simulink model "model1"  (R2023a)
settings: Solver=ode4  StartTime=0.0  StopTime=500  FixedStep=simulation_dt  RelTol=1e-3
undefined symbols (not defined in the file or in its folder): input, k_harmonics, magnitude, simulation_dt
libraries: simulink x3
settings Model: Creator=dionl  LastModifiedBy=dionl

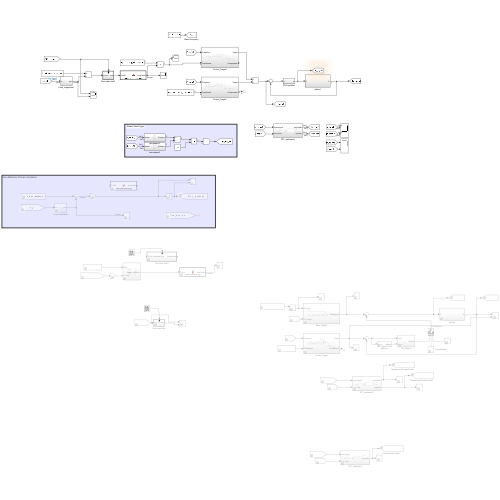
[thumbnail: Simulink's stored preview of the top-level diagram]
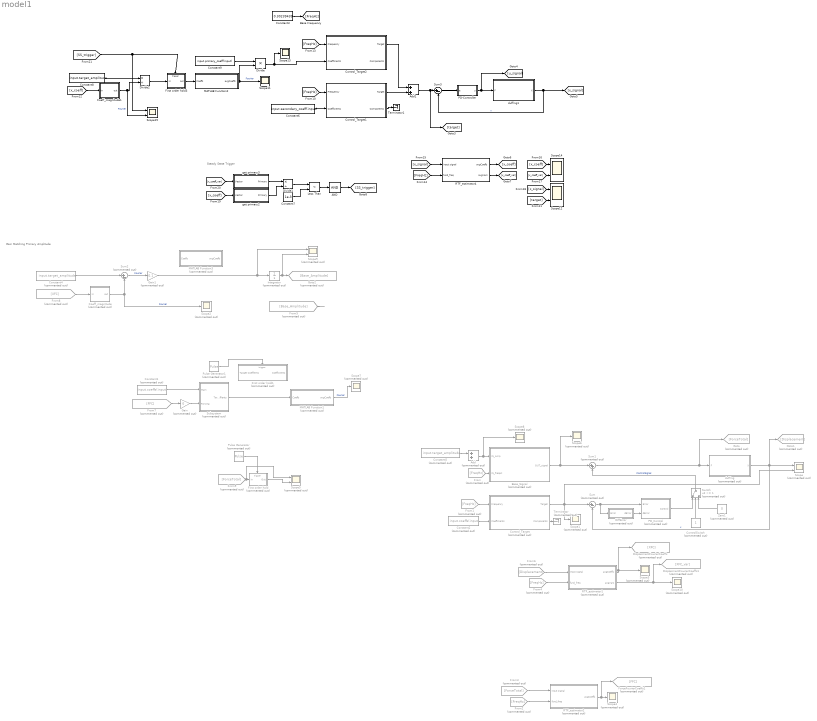
== system model1 ==
  note: Steady State Trigger
  note: Gain Matching Primary Amplitude
  AND : Logic  Inputs=1  IconShape=distinctive  AllPortsSameDT=off  OutDataTypeStr=boolean
  Add : Sum  Commented=on
  Add1 : Sum
  Base_Signal : Subsystem  Commented=on
  Coeff_magnitude : Subsystem  Commented=on
  Coeff_magnitude1 : Subsystem
  Constant1 : Constant  Commented=on  Value=input.coeffs(input)
  Constant2 : Constant  Commented=on  Value=input.coeffs(input)
  Constant3 : Constant  Value=0.30239439
  Constant4 : Constant  Commented=on  Value=input.target_amplitude
  Constant5 : Constant  Commented=on  Value=input.target_amplitude
  Constant6 : Constant  Value=input.secondary_coeff(input)
  Constant7 : Constant  Value=1e-3
  Constant8 : Constant  Value=input.target_amplitude
  Constant9 : Constant  Value=input.primary_coeff(input)
  ControlSwitch : Constant  Commented=on
  Control_Target : Subsystem  Commented=on
  Control_Target1 : Subsystem
  Control_Target2 : Subsystem
  DiffError : Subsystem  Commented=on
  DisplacmentFourierCoeffs : Goto  Commented=on  GotoTag=XFC
  DisplacmentFourierCoeffs1 : Goto  Commented=on  GotoTag=XFC_var
  Divide : Product  Inputs=**
  Divide1 : Product  Inputs=*/
  Divide2 : Product  Inputs=*/
  First order hold : Subsystem  Commented=on  TreatAsAtomicUnit=on
  First order hold1 : Subsystem  Commented=on  TreatAsAtomicUnit=on
  First order hold3 : Subsystem  TreatAsAtomicUnit=on
  ForceFourierCoeffs1 : Goto  Commented=on  GotoTag=FFC
  From{,1..2,4} (4 alike) : From  Commented=on  GotoTag=FreqHz
  From3 : From  Commented=on  GotoTag=ForceTotal
  From5 : From  Commented=on  GotoTag=Base_Amplitude
  From6 : From  Commented=on  GotoTag=Displacement
  From7 : From  Commented=on  GotoTag=FFC
  From8 : From  Commented=on  GotoTag=XFC
  From9 : From  Commented=on  GotoTag=ForceTotal
  Gain : Gain  Commented=on  Gain=0
  Gain1 : Gain  Commented=on  Gain=0.1
  Goto : Goto  Commented=on  GotoTag=ForceTotal
  Goto1 : Goto  Commented=on  GotoTag=Displacement
  Goto2 : Goto  Commented=on  GotoTag=Base_Amplitude
  Integrator : Integrator  Commented=on
  Less Than : RelationalOperator  Operator=<  OutDataTypeStr=boolean  RndMeth=Simplest  InputSameDT=off
  MATLAB Function1 : MATLAB Function  Commented=on  TreatAsAtomicUnit=on
  MATLAB Function2 : MATLAB Function  TreatAsAtomicUnit=on
  MATLAB Function3 : MATLAB Function  Commented=on  TreatAsAtomicUnit=on
  PD-Controller : Subsystem
  PD_Control : Subsystem  Commented=on
  Pulse Generator : DiscretePulseGenerator  Commented=on  PulseType=Time based  Period=1  PulseWidth=5
  Pulse Generator1 : DiscretePulseGenerator  Commented=on  PulseType=Time based  Period=100  PulseWidth=5  PhaseDelay=simulation_dt
  RTF_estimator1 : Subsystem  Commented=on
  RTF_estimator2 : Subsystem  Commented=on
  RTF_estimator4 : Subsystem
  Scope : Scope  Commented=on  NumInputPorts=2
  Scope{1..4,6..8,10} (8 alike) : Scope  Commented=on
  Scope11 : Scope
  Scope12 : Scope  NumInputPorts=2
  Scope13 : Scope
  Scope14 : Scope  NumInputPorts=2
  Scope15 : Scope  NumInputPorts=2
  Scope5 : Scope  Commented=on  NumInputPorts=2
  Scope9 : Scope  Commented=on  NumInputPorts=2
  Subsystem : Subsystem  Commented=on
  Sum : Sum  Commented=on  Inputs=|+-
  Sum1 : Sum  Commented=on  Inputs=|++
  Sum2 : Sum  Commented=on  Inputs=|+-
  Sum3 : Sum  Inputs=|+-
  Switch : Switch  Commented=on  Threshold=1  SaturateOnIntegerOverflow=off  InputSameDT=off
  Terminator : Terminator  Commented=on
  Terminator1 : Terminator
  Zero1 : Constant  Commented=on  Value=0
  duffing : Subsystem  Commented=on
  duffing1 : Subsystem
  get primary2 : Subsystem
  get primary3 : Subsystem
  wires:
  From/1 -> Base_Signal/2(IN_freqHz)
  Base_Signal/1(OUT_signal) -> Scope6/1, Sum1/1
  Control_Target/1(Target) -> Scope1/1, Scope/2, Sum/1
  duffing/1(X) -> Goto1/1, Scope/1, Sum/2  "x"
  Sum/1 -> DiffError/1(Error), PD_Control/1(Error)
  DiffError/1(dError) -> PD_Control/2(dError)
  Switch/1 -> Sum1/2  "ControlSignal"
  ControlSwitch/1 -> Switch/2
  Zero1/1 -> Switch/3
  PD_Control/1(Control) -> Switch/1
  Sum1/1 -> Goto/1, duffing/1(F)
  Constant3/1 -> [FreqHz]
  From1/1 -> Control_Target/1(Frequency)
  From4/1 -> RTF_estimator1/2(fund_freq)
  RTF_estimator1/1(avgCoeffs) -> Scope3/1, DisplacmentFourierCoeffs/1
  RTF_estimator2/1(avgCoeffs) -> ForceFourierCoeffs1/1, Scope4/1
  From2/1 -> RTF_estimator2/2(fund_freq)
  From3/1 -> RTF_estimator2/1(input signal)
  Control_Target/2(Components) -> Terminator/1
  From6/1 -> RTF_estimator1/1(input signal)
  Sum2/1 -> Gain1/1  "Fourier"
  From8/1 -> Coeff_magnitude/1(in)
  Integrator/1 -> Scope9/2, Goto2/1
  Constant4/1 -> Sum2/1
  Pulse Generator/1 -> First order hold/Trigger
  From9/1 -> Scope5/1, First order hold/1(In)
  First order hold/1(Out) -> Scope5/2
  Constant1/1 -> Subsystem/1(Main)
  From7/1 -> Gain/1
  Subsystem/1(Target Coeffients) -> MATLAB Function1/1(Coeffs)
  Pulse Generator1/1 -> First order hold1/Trigger
  Gain/1 -> Subsystem/2(Forcing)
  MATLAB Function1/1(avgCoeffs) -> Scope7/1  "Fourier"
  Constant2/1 -> Control_Target/2(Coefficients)
  From5/1 -> ?
  Constant5/1 -> Add/1
  Add/1 -> Scope8/1, Base_Signal/1(IN_Amp)
  RTF_estimator1/2(avgVars) -> DisplacmentFourierCoeffs1/1, Scope10/1
  Coeff_magnitude/1(out) -> Scope2/1, Sum2/2  "Fourier"
  Gain1/1 -> Scope9/1, Integrator/1
  [FreqHz] -> Control_Target1/1(Frequency)
  Control_Target1/2(Components) -> Terminator1/1
  Control_Target1/1(Target) -> Add1/2
  Sum3/1 -> PD-Controller/1(e)
  duffing1/1(X) -> [x_signal], Sum3/2  "x"
  PD-Controller/1(u) -> [u_signal], duffing1/1(F)
  [target] -> Scope12/2
  [x_signal] -> RTF_estimator4/1(input signal)
  [FreqHz] -> RTF_estimator4/2(fund_freq)
  RTF_estimator4/1(avgCoeffs) -> [x_coeff]
  RTF_estimator4/2(avgVars) -> [x_coeff_var]
  [x_coeff_var] -> Scope14/2
  [x_coeff] -> Scope14/1
  [x_signal] -> Scope12/1
  [x_coeff] -> get primary2/1(Vector)
  [x_coeff_var] -> get primary3/1(Vector)
  get primary3/1(Primary) -> Divide1/1
  get primary2/1(Primary) -> Divide1/2
  Divide1/1 -> Less Than/1
  Constant7/1 -> Less Than/2
  Less Than/1 -> AND/1
  AND/1 -> [SS_trigger]
  [SS_trigger] -> First order hold3/Trigger, Scope15/1
  [x_coeff] -> Coeff_magnitude1/1(in)
  Constant8/1 -> Divide2/1
  Coeff_magnitude1/1(out) -> Scope15/2, Divide2/2  "Fourier"
  Constant6/1 -> Control_Target1/2(Coefficients)
  [FreqHz] -> Control_Target2/1(Frequency)
  Control_Target2/1(Target) -> Add1/1
  Add1/1 -> [target], Sum3/1
  Constant9/1 -> Divide/1
  Divide/1 -> Scope13/1, Control_Target2/2(Coefficients)
  First order hold3/1(out) -> MATLAB Function2/1(Coeffs)
  Divide2/1 -> First order hold3/1(in)
  MATLAB Function2/1(avgCoeffs) -> Divide/2, Scope11/1  "Fourier"

== system model1/Base_Signal ==
  IN_Amp : Inport
  IN_freqHz : Inport  Port=2
  Gain : Gain  Gain=2*pi
  Integrator : Integrator
  Product : Product
  Sin : Trigonometry
  OUT_signal : Outport
  wires:
  IN_Amp/1 -> Product/1
  Integrator/1 -> Gain/1
  Gain/1 -> Sin/1
  IN_freqHz/1 -> Integrator/1
  Sin/1 -> Product/2
  Product/1 -> OUT_signal/1

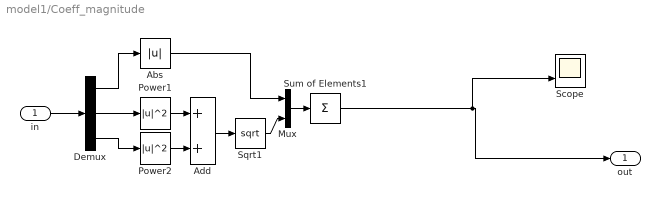
== system model1/Coeff_magnitude ==
  in : Inport
  Abs : Abs  SaturateOnIntegerOverflow=off
  Add : Sum
  Demux : Demux  Outputs=[1 k_harmonics k_harmonics]
  Mux : Mux  Inputs=2
  Power1 : Math  Operator=magnitude^2
  Power2 : Math  Operator=magnitude^2
  Scope : Scope  NumInputPorts=2
  Sqrt1 : Sqrt
  Sum of Elements1 : Sum  Inputs=+
  out : Outport
  wires:
  in/1 -> Demux/1
  Demux/1 -> Abs/1
  Demux/2 -> Power1/1
  Demux/3 -> Power2/1
  Power1/1 -> Add/1
  Power2/1 -> Add/2
  Add/1 -> Sqrt1/1
  Abs/1 -> Mux/1
  Sqrt1/1 -> Mux/2
  Mux/1 -> Sum of Elements1/1
  Sum of Elements1/1 -> Scope/2, out/1

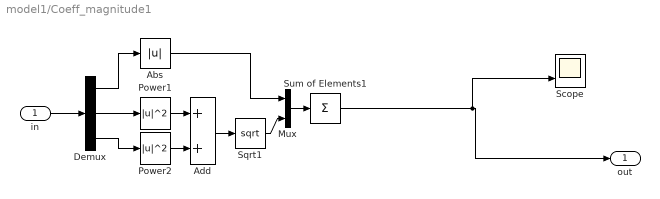
== system model1/Coeff_magnitude1 ==
  in : Inport
  Abs : Abs  SaturateOnIntegerOverflow=off
  Add : Sum
  Demux : Demux  Outputs=[1 k_harmonics k_harmonics]
  Mux : Mux  Inputs=2
  Power1 : Math  Operator=magnitude^2
  Power2 : Math  Operator=magnitude^2
  Scope : Scope  NumInputPorts=2
  Sqrt1 : Sqrt
  Sum of Elements1 : Sum  Inputs=+
  out : Outport
  wires:
  in/1 -> Demux/1
  Demux/1 -> Abs/1
  Demux/2 -> Power1/1
  Demux/3 -> Power2/1
  Power1/1 -> Add/1
  Power2/1 -> Add/2
  Add/1 -> Sqrt1/1
  Abs/1 -> Mux/1
  Sqrt1/1 -> Mux/2
  Mux/1 -> Sum of Elements1/1
  Sum of Elements1/1 -> Scope/2, out/1

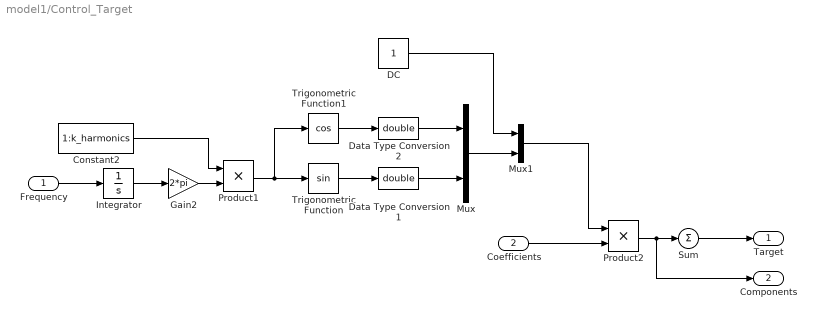
== system model1/Control_Target ==
  Frequency : Inport
  Coefficients : Inport  Port=2
  Constant2 : Constant  Value=1:k_harmonics
  DC : Constant
  Data Type Conversion1 : DataTypeConversion  OutDataTypeStr=double  SaturateOnIntegerOverflow=off  RndMeth=Floor
  Data Type Conversion2 : DataTypeConversion  OutDataTypeStr=double  SaturateOnIntegerOverflow=off  RndMeth=Floor
  Gain2 : Gain  Gain=2*pi
  Integrator : Integrator
  Mux : Mux  Inputs=2
  Mux1 : Mux  Inputs=2
  Product1 : Product
  Product2 : Product  RndMeth=Zero
  Sum : Sum  Inputs=|+|
  Trigonometric Function : Trigonometry
  Trigonometric Function1 : Trigonometry  Operator=cos
  Target : Outport
  Components : Outport  Port=2
  wires:
  Data Type Conversion1/1 -> Mux/2
  Product1/1 -> Trigonometric Function1/1, Trigonometric Function/1
  Gain2/1 -> Product1/2
  Frequency/1 -> Integrator/1
  Constant2/1 -> Product1/1
  Coefficients/1 -> Product2/2
  Product2/1 -> Components/1, Sum/1
  Mux1/1 -> Product2/1
  DC/1 -> Mux1/1
  Trigonometric Function1/1 -> Data Type Conversion2/1
  Data Type Conversion2/1 -> Mux/1
  Trigonometric Function/1 -> Data Type Conversion1/1
  Mux/1 -> Mux1/2
  Integrator/1 -> Gain2/1
  Sum/1 -> Target/1

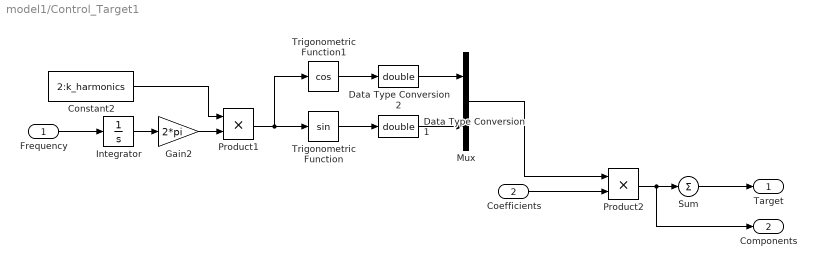
== system model1/Control_Target1 ==
  Frequency : Inport
  Coefficients : Inport  Port=2
  Constant2 : Constant  Value=2:k_harmonics
  Data Type Conversion1 : DataTypeConversion  OutDataTypeStr=double  SaturateOnIntegerOverflow=off  RndMeth=Floor
  Data Type Conversion2 : DataTypeConversion  OutDataTypeStr=double  SaturateOnIntegerOverflow=off  RndMeth=Floor
  Gain2 : Gain  Gain=2*pi
  Integrator : Integrator
  Mux : Mux  Inputs=2
  Product1 : Product
  Product2 : Product  RndMeth=Zero
  Sum : Sum  Inputs=|+|
  Trigonometric Function : Trigonometry
  Trigonometric Function1 : Trigonometry  Operator=cos
  Target : Outport
  Components : Outport  Port=2
  wires:
  Sum/1 -> Target/1
  Integrator/1 -> Gain2/1
  Trigonometric Function/1 -> Data Type Conversion1/1
  Data Type Conversion2/1 -> Mux/1
  Trigonometric Function1/1 -> Data Type Conversion2/1
  Mux/1 -> Product2/1
  Product2/1 -> Sum/1, Components/1
  Coefficients/1 -> Product2/2
  Constant2/1 -> Product1/1
  Frequency/1 -> Integrator/1
  Gain2/1 -> Product1/2
  Product1/1 -> Trigonometric Function/1, Trigonometric Function1/1
  Data Type Conversion1/1 -> Mux/2

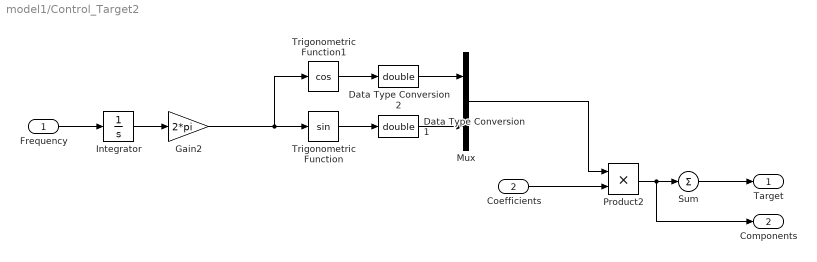
== system model1/Control_Target2 ==
  Frequency : Inport
  Coefficients : Inport  Port=2
  Data Type Conversion1 : DataTypeConversion  OutDataTypeStr=double  SaturateOnIntegerOverflow=off  RndMeth=Floor
  Data Type Conversion2 : DataTypeConversion  OutDataTypeStr=double  SaturateOnIntegerOverflow=off  RndMeth=Floor
  Gain2 : Gain  Gain=2*pi
  Integrator : Integrator
  Mux : Mux  Inputs=2
  Product2 : Product  RndMeth=Zero
  Sum : Sum  Inputs=|+|
  Trigonometric Function : Trigonometry
  Trigonometric Function1 : Trigonometry  Operator=cos
  Target : Outport
  Components : Outport  Port=2
  wires:
  Data Type Conversion1/1 -> Mux/2
  Gain2/1 -> Trigonometric Function1/1, Trigonometric Function/1
  Frequency/1 -> Integrator/1
  Coefficients/1 -> Product2/2
  Product2/1 -> Components/1, Sum/1
  Mux/1 -> Product2/1
  Trigonometric Function1/1 -> Data Type Conversion2/1
  Data Type Conversion2/1 -> Mux/1
  Trigonometric Function/1 -> Data Type Conversion1/1
  Integrator/1 -> Gain2/1
  Sum/1 -> Target/1

== system model1/DiffError ==
  Error : Inport
  Sum4 : Sum  Inputs=|-+
  Unit Delay : UnitDelay  SampleTime=-1  HasFrameUpgradeWarning=on
  Weighted Sample Time : SampleTimeMath  TsampMathOp=/
  dError : Outport
  wires:
  Unit Delay/1 -> Sum4/1
  Sum4/1 -> Weighted Sample Time/1
  Weighted Sample Time/1 -> dError/1
  Error/1 -> Unit Delay/1, Sum4/2

== system model1/First order hold ==
  In : Inport  LatchByDelayingOutsideSignal=on
  Trigger : TriggerPort  VariantControl=(inherit)
  Out : Outport
  wires:
  In/1 -> Out/1

== system model1/First order hold1 ==
  Target Coeffients : Inport  LatchByDelayingOutsideSignal=on
  Trigger : TriggerPort  VariantControl=(inherit)
  Coefficients : Outport
  wires:
  Target Coeffients/1 -> Coefficients/1

== system model1/First order hold3 ==
  in : Inport  LatchByDelayingOutsideSignal=on
  Trigger : TriggerPort  VariantControl=(inherit)
  out : Outport  InitialOutput=1
  wires:
  in/1 -> out/1

== system model1/PD-Controller ==
  e : Inport
  Add1 : Sum
  DiffError1 : Subsystem
  Kd : Gain
  Kp : Gain  Gain=2
  u : Outport
  wires:
  DiffError1/1(dError) -> Kd/1
  Kp/1 -> Add1/1
  e/1 -> DiffError1/1(Error), Kp/1
  Kd/1 -> Add1/2
  Add1/1 -> u/1

== system model1/PD_Control ==
  Error : Inport
  dError : Inport  Port=2
  Kd : Constant
  Kp : Constant  Value=2
  Product : Product  RndMeth=Zero
  Product1 : Product  RndMeth=Zero
  Sum2 : Sum  Inputs=+|+
  Control : Outport
  wires:
  Kp/1 -> Product/1
  Kd/1 -> Product1/2
  Product/1 -> Sum2/1
  Product1/1 -> Sum2/2
  Error/1 -> Product/2
  Sum2/1 -> Control/1  "Control"
  dError/1 -> Product1/1

== system model1/RTF_estimator1 ==
  input signal : Inport
  fund_freq : Inport  Port=2
  MATLAB Function1 : MATLAB Function  TreatAsAtomicUnit=on
  Subsystem : Subsystem
  Terminator : Terminator
  avgCoeffs : Outport
  avgVars : Outport  Port=2
  wires:
  input signal/1 -> Subsystem/1(input signal)
  Subsystem/2(Phase1) -> Terminator/1
  fund_freq/1 -> Subsystem/2(fund_freq)
  Subsystem/1(Fourier1) -> MATLAB Function1/1(Coeffs)
  MATLAB Function1/2(varCoeffs) -> avgVars/1
  MATLAB Function1/1(avgCoeffs) -> avgCoeffs/1  "Fourier"

== system model1/RTF_estimator2 ==
  input signal : Inport
  fund_freq : Inport  Port=2
  MATLAB Function2 : MATLAB Function  TreatAsAtomicUnit=on
  MATLAB Function3 : MATLAB Function  Commented=on  TreatAsAtomicUnit=on
  Subsystem : Subsystem
  Terminator : Terminator
  avgCoeffs : Outport
  wires:
  Subsystem/1(Fourier1) -> MATLAB Function2/1(Coeffs)
  MATLAB Function2/1(avgCoeffs) -> avgCoeffs/1  "Fourier"
  fund_freq/1 -> Subsystem/2(fund_freq)
  Subsystem/2(Phase1) -> Terminator/1
  input signal/1 -> Subsystem/1(input signal)

== system model1/RTF_estimator4 ==
  input signal : Inport
  fund_freq : Inport  Port=2
  MATLAB Function1 : MATLAB Function  TreatAsAtomicUnit=on
  Subsystem : Subsystem
  Terminator : Terminator
  avgCoeffs : Outport
  avgVars : Outport  Port=2
  wires:
  input signal/1 -> Subsystem/1(input signal)
  Subsystem/2(Phase1) -> Terminator/1
  fund_freq/1 -> Subsystem/2(fund_freq)
  Subsystem/1(Fourier1) -> MATLAB Function1/1(Coeffs)
  MATLAB Function1/2(varCoeffs) -> avgVars/1
  MATLAB Function1/1(avgCoeffs) -> avgCoeffs/1  "Fourier"

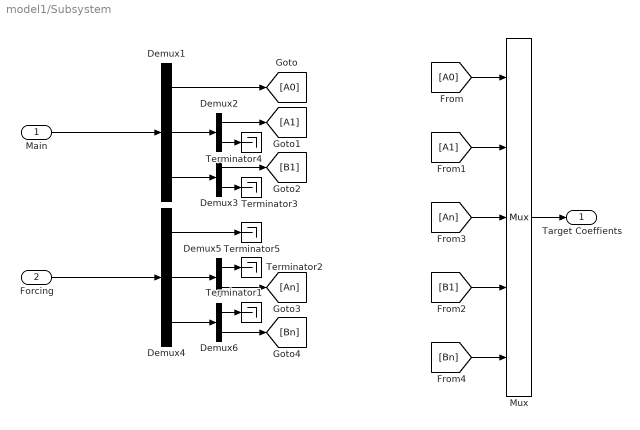
== system model1/Subsystem ==
  Main : Inport
  Forcing : Inport  Port=2
  Demux1 : Demux  Outputs=[1 k_harmonics k_harmonics]
  Demux{2..3,5..6} (4 alike) : Demux  Outputs=[1 -1]
  Demux4 : Demux  Outputs=[1 k_harmonics k_harmonics]
  Mux : Mux  Inputs=5
  Terminator{1..5} (5 alike) : Terminator
  Target Coeffients : Outport
  wires:
  Demux1/3 -> Demux3/1
  Demux4/3 -> Demux6/1
  Forcing/1 -> Demux4/1
  Demux2/2 -> Terminator4/1
  Main/1 -> Demux1/1
  Demux5/1 -> Terminator2/1
  Demux6/1 -> Terminator1/1
  Demux4/2 -> Demux5/1
  Demux4/1 -> Terminator5/1
  Demux3/2 -> Terminator3/1
  Demux1/2 -> Demux2/1
  Mux/1 -> Target Coeffients/1
  Demux1/1 -> [A0]
  [A0] -> Mux/1
  Demux2/1 -> [A1]
  [A1] -> Mux/2
  Demux3/1 -> [B1]
  Demux5/2 -> [An]
  Demux6/2 -> [Bn]
  [An] -> Mux/3
  [B1] -> Mux/4
  [Bn] -> Mux/5

== system model1/duffing ==
  F : Inport
  Integrator : Integrator
  Integrator1 : Integrator
  MATLAB Function : MATLAB Function  TreatAsAtomicUnit=on
  X : Outport
  wires:
  Integrator1/1 -> MATLAB Function/2(v)
  MATLAB Function/2(dvdt) -> Integrator1/1
  MATLAB Function/1(dxdt) -> Integrator/1
  F/1 -> MATLAB Function/3(excitation)
  Integrator/1 -> MATLAB Function/1(x), X/1

== system model1/duffing1 ==
  F : Inport
  Integrator : Integrator
  Integrator1 : Integrator
  MATLAB Function : MATLAB Function  TreatAsAtomicUnit=on
  X : Outport
  wires:
  Integrator/1 -> X/1, MATLAB Function/1(x)
  F/1 -> MATLAB Function/3(excitation)
  MATLAB Function/1(dxdt) -> Integrator/1
  MATLAB Function/2(dvdt) -> Integrator1/1
  Integrator1/1 -> MATLAB Function/2(v)

== system model1/get primary2 ==
  Vector : Inport
  Demux : Demux  Outputs=[1, 1, k_harmonics-1, 1, k_harmonics-1]
  Mux : Mux  Inputs=2
  Terminator2 : Terminator
  Terminator3 : Terminator
  Terminator4 : Terminator
  Primary : Outport
  wires:
  Vector/1 -> Demux/1
  Demux/5 -> Terminator4/1
  Demux/3 -> Terminator3/1
  Mux/1 -> Primary/1
  Demux/4 -> Mux/2
  Demux/2 -> Mux/1
  Demux/1 -> Terminator2/1

== system model1/get primary3 ==
  Vector : Inport
  Demux : Demux  Outputs=[1, 1, k_harmonics-1, 1, k_harmonics-1]
  Mux : Mux  Inputs=2
  Terminator2 : Terminator
  Terminator3 : Terminator
  Terminator4 : Terminator
  Primary : Outport
  wires:
  Demux/1 -> Terminator2/1
  Demux/2 -> Mux/1
  Demux/4 -> Mux/2
  Mux/1 -> Primary/1
  Demux/3 -> Terminator3/1
  Demux/5 -> Terminator4/1
  Vector/1 -> Demux/1

== system model1/PD-Controller/DiffError1 ==
  Error : Inport
  Sum4 : Sum  Inputs=|-+
  Unit Delay : UnitDelay  SampleTime=-1  HasFrameUpgradeWarning=on
  Weighted Sample Time : SampleTimeMath  TsampMathOp=/
  dError : Outport
  wires:
  Unit Delay/1 -> Sum4/1
  Sum4/1 -> Weighted Sample Time/1
  Weighted Sample Time/1 -> dError/1
  Error/1 -> Unit Delay/1, Sum4/2

== system model1/RTF_estimator1/Subsystem ==
  input signal : Inport
  fund_freq : Inport  Port=2
  Fourier Series 2 : Subsystem
  Harmonic Basis Gen1 : Subsystem
  Fourier1 : Outport
  Phase1 : Outport  Port=2
  wires:
  Fourier Series 2/2(Phase) -> Phase1/1
  input signal/1 -> Fourier Series 2/1(input signal)
  Fourier Series 2/1(Fourier) -> Fourier1/1
  fund_freq/1 -> Harmonic Basis Gen1/1(fund_freq), Fourier Series 2/3(fundamental frequency)
  Harmonic Basis Gen1/1(harmonic_basis) -> Fourier Series 2/2(harmonic basis)

== system model1/RTF_estimator2/Subsystem ==
  input signal : Inport
  fund_freq : Inport  Port=2
  Fourier Series 2 : Subsystem
  Harmonic Basis Gen1 : Subsystem
  Fourier1 : Outport
  Phase1 : Outport  Port=2
  wires:
  Harmonic Basis Gen1/1(harmonic_basis) -> Fourier Series 2/2(harmonic basis)
  fund_freq/1 -> Fourier Series 2/3(fundamental frequency), Harmonic Basis Gen1/1(fund_freq)
  Fourier Series 2/1(Fourier) -> Fourier1/1
  input signal/1 -> Fourier Series 2/1(input signal)
  Fourier Series 2/2(Phase) -> Phase1/1

== system model1/RTF_estimator4/Subsystem ==
  input signal : Inport
  fund_freq : Inport  Port=2
  Fourier Series 2 : Subsystem
  Harmonic Basis Gen1 : Subsystem
  Fourier1 : Outport
  Phase1 : Outport  Port=2
  wires:
  Fourier Series 2/2(Phase) -> Phase1/1
  input signal/1 -> Fourier Series 2/1(input signal)
  Fourier Series 2/1(Fourier) -> Fourier1/1
  fund_freq/1 -> Harmonic Basis Gen1/1(fund_freq), Fourier Series 2/3(fundamental frequency)
  Harmonic Basis Gen1/1(harmonic_basis) -> Fourier Series 2/2(harmonic basis)

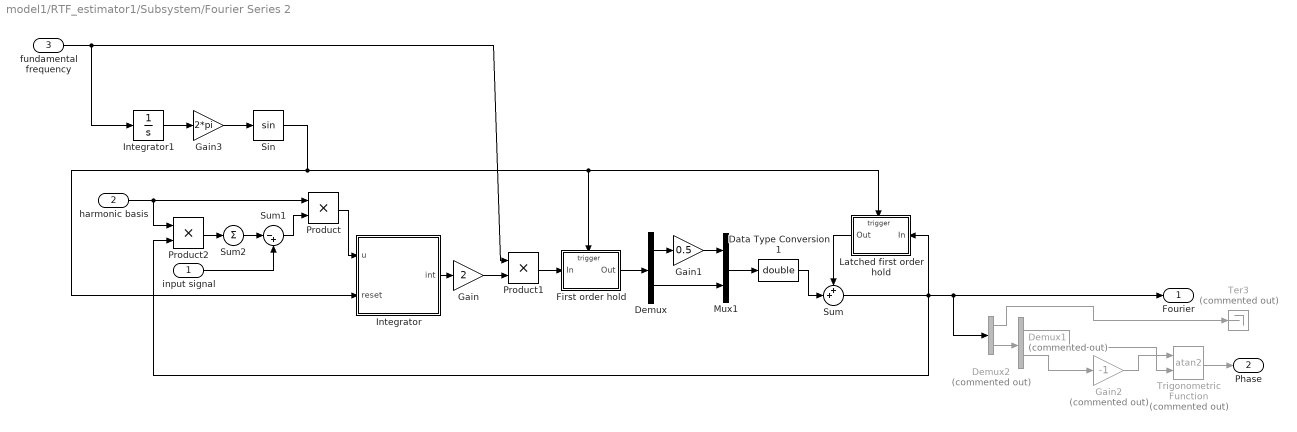
== system model1/RTF_estimator1/Subsystem/Fourier Series 2 ==
  input signal : Inport
  harmonic basis : Inport  Port=2
  fundamental frequency : Inport  Port=3
  Data Type Conversion1 : DataTypeConversion  OutDataTypeStr=double  SaturateOnIntegerOverflow=off  RndMeth=Floor
  Demux : Demux  Outputs=[1 -1]
  Demux1 : Demux  Commented=on  Outputs=2
  Demux2 : Demux  Commented=on  Outputs=[1 -1]
  First order hold : Subsystem  TreatAsAtomicUnit=on
  Gain : Gain  Gain=2
  Gain1 : Gain  Gain=0.5
  Gain2 : Gain  Commented=on  Gain=-1
  Gain3 : Gain  Gain=2*pi
  Integrator : Subsystem
  Integrator1 : Integrator
  Latched first order hold : Subsystem  TreatAsAtomicUnit=on
  Mux1 : Mux  Inputs=2
  Product : Product  RndMeth=Zero
  Product1 : Product  RndMeth=Zero
  Product2 : Product  RndMeth=Zero
  Sin : Trigonometry
  Sum : Sum  Tag=Test  Inputs=++|
  Sum1 : Sum  Inputs=|-+
  Sum2 : Sum  Inputs=|+|
  Ter3 : Terminator  Commented=on
  Trigonometric Function : Trigonometry  Commented=on  Operator=atan2
  Fourier : Outport
  Phase : Outport  Port=2
  wires:
  fundamental frequency/1 -> Product1/1, Integrator1/1
  Integrator1/1 -> Gain3/1
  Gain3/1 -> Sin/1
  Demux2/1 -> Ter3/1
  Demux2/2 -> Demux1/1
  Gain2/1 -> Trigonometric Function/1
  Demux1/2 -> Gain2/1
  Demux1/1 -> Trigonometric Function/2
  Product/1 -> Integrator/1(u)
  Trigonometric Function/1 -> Phase/1
  Sum2/1 -> Sum1/1
  harmonic basis/1 -> Product2/1, Product/1
  input signal/1 -> Sum1/2
  Product2/1 -> Sum2/1
  Sum1/1 -> Product/2
  Latched first order hold/1(Out) -> Sum/1
  Sum/1 -> Demux2/1, Fourier/1, Latched first order hold/1(In), Product2/2
  Data Type Conversion1/1 -> Sum/2
  Mux1/1 -> Data Type Conversion1/1
  First order hold/1(Out) -> Demux/1
  Demux/2 -> Mux1/2
  Gain1/1 -> Mux1/1
  Demux/1 -> Gain1/1
  Integrator/1(int) -> Gain/1
  Sin/1 -> Latched first order hold/Trigger, First order hold/Trigger, Integrator/2(reset)
  Gain/1 -> Product1/2
  Product1/1 -> First order hold/1(In)

== system model1/RTF_estimator1/Subsystem/Harmonic Basis Gen1 ==
  fund_freq : Inport
  Cos : Trigonometry  Operator=cos
  DC : Constant
  Gain1 : Gain  Gain=2*pi
  Integrator : Integrator
  Mux : Mux  Inputs=3
  Product : Product
  Sin : Trigonometry
  harmonics_array : Constant  Value=1:k_harmonics
  harmonic_basis : Outport  OutDataTypeStr=double  SampleTime=0
  wires:
  Gain1/1 -> Sin/1, Cos/1
  Mux/1 -> harmonic_basis/1
  Integrator/1 -> Product/1
  Cos/1 -> Mux/2
  Product/1 -> Gain1/1
  Sin/1 -> Mux/3
  harmonics_array/1 -> Product/2
  fund_freq/1 -> Integrator/1
  DC/1 -> Mux/1

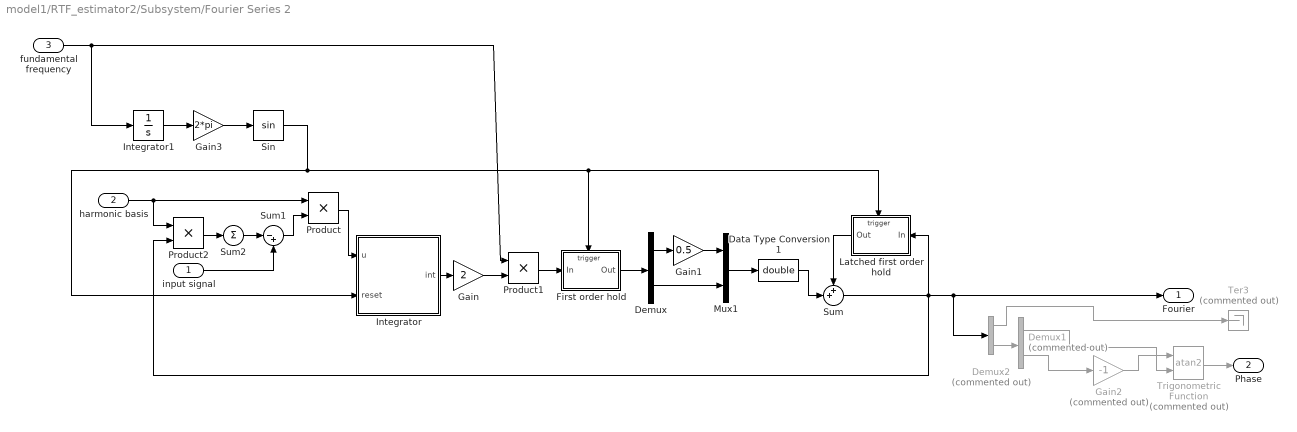
== system model1/RTF_estimator2/Subsystem/Fourier Series 2 ==
  input signal : Inport
  harmonic basis : Inport  Port=2
  fundamental frequency : Inport  Port=3
  Data Type Conversion1 : DataTypeConversion  OutDataTypeStr=double  SaturateOnIntegerOverflow=off  RndMeth=Floor
  Demux : Demux  Outputs=[1 -1]
  Demux1 : Demux  Commented=on  Outputs=2
  Demux2 : Demux  Commented=on  Outputs=[1 -1]
  First order hold : Subsystem  TreatAsAtomicUnit=on
  Gain : Gain  Gain=2
  Gain1 : Gain  Gain=0.5
  Gain2 : Gain  Commented=on  Gain=-1
  Gain3 : Gain  Gain=2*pi
  Integrator : Subsystem
  Integrator1 : Integrator
  Latched first order hold : Subsystem  TreatAsAtomicUnit=on
  Mux1 : Mux  Inputs=2
  Product : Product  RndMeth=Zero
  Product1 : Product  RndMeth=Zero
  Product2 : Product  RndMeth=Zero
  Sin : Trigonometry
  Sum : Sum  Tag=Test  Inputs=++|
  Sum1 : Sum  Inputs=|-+
  Sum2 : Sum  Inputs=|+|
  Ter3 : Terminator  Commented=on
  Trigonometric Function : Trigonometry  Commented=on  Operator=atan2
  Fourier : Outport
  Phase : Outport  Port=2
  wires:
  Product1/1 -> First order hold/1(In)
  Gain/1 -> Product1/2
  Sin/1 -> Integrator/2(reset), First order hold/Trigger, Latched first order hold/Trigger
  Integrator/1(int) -> Gain/1
  Demux/1 -> Gain1/1
  Gain1/1 -> Mux1/1
  Demux/2 -> Mux1/2
  First order hold/1(Out) -> Demux/1
  Mux1/1 -> Data Type Conversion1/1
  Data Type Conversion1/1 -> Sum/2
  Sum/1 -> Product2/2, Latched first order hold/1(In), Fourier/1, Demux2/1
  Latched first order hold/1(Out) -> Sum/1
  Sum1/1 -> Product/2
  Product2/1 -> Sum2/1
  input signal/1 -> Sum1/2
  harmonic basis/1 -> Product/1, Product2/1
  Sum2/1 -> Sum1/1
  Trigonometric Function/1 -> Phase/1
  Product/1 -> Integrator/1(u)
  Demux1/1 -> Trigonometric Function/2
  Demux1/2 -> Gain2/1
  Gain2/1 -> Trigonometric Function/1
  Demux2/2 -> Demux1/1
  Demux2/1 -> Ter3/1
  Gain3/1 -> Sin/1
  Integrator1/1 -> Gain3/1
  fundamental frequency/1 -> Integrator1/1, Product1/1

== system model1/RTF_estimator2/Subsystem/Harmonic Basis Gen1 ==
  fund_freq : Inport
  Cos : Trigonometry  Operator=cos
  DC : Constant
  Gain1 : Gain  Gain=2*pi
  Integrator : Integrator
  Mux : Mux  Inputs=3
  Product : Product
  Sin : Trigonometry
  harmonics_array : Constant  Value=1:k_harmonics
  harmonic_basis : Outport  OutDataTypeStr=double  SampleTime=0
  wires:
  DC/1 -> Mux/1
  fund_freq/1 -> Integrator/1
  harmonics_array/1 -> Product/2
  Sin/1 -> Mux/3
  Product/1 -> Gain1/1
  Cos/1 -> Mux/2
  Integrator/1 -> Product/1
  Mux/1 -> harmonic_basis/1
  Gain1/1 -> Cos/1, Sin/1

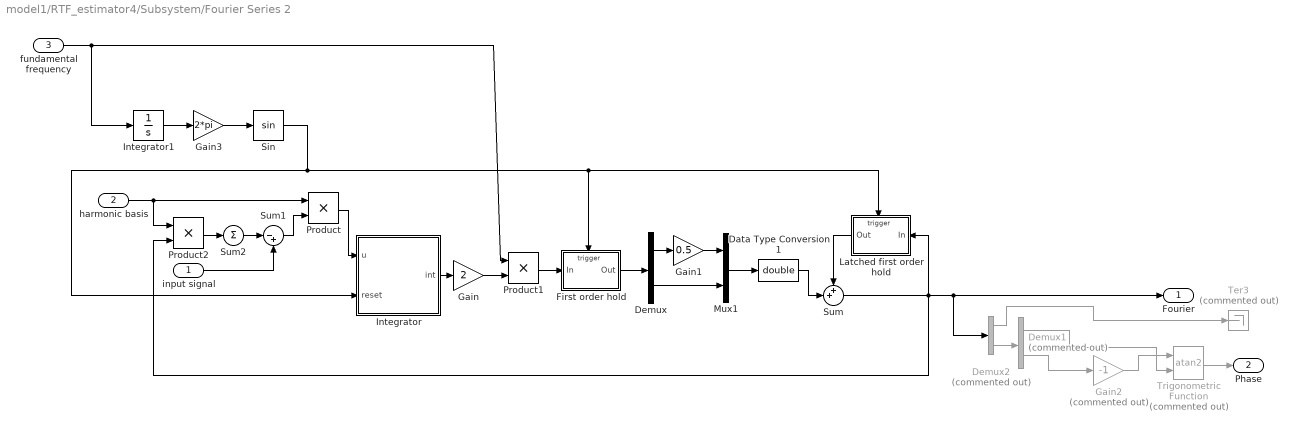
== system model1/RTF_estimator4/Subsystem/Fourier Series 2 ==
  input signal : Inport
  harmonic basis : Inport  Port=2
  fundamental frequency : Inport  Port=3
  Data Type Conversion1 : DataTypeConversion  OutDataTypeStr=double  SaturateOnIntegerOverflow=off  RndMeth=Floor
  Demux : Demux  Outputs=[1 -1]
  Demux1 : Demux  Commented=on  Outputs=2
  Demux2 : Demux  Commented=on  Outputs=[1 -1]
  First order hold : Subsystem  TreatAsAtomicUnit=on
  Gain : Gain  Gain=2
  Gain1 : Gain  Gain=0.5
  Gain2 : Gain  Commented=on  Gain=-1
  Gain3 : Gain  Gain=2*pi
  Integrator : Subsystem
  Integrator1 : Integrator
  Latched first order hold : Subsystem  TreatAsAtomicUnit=on
  Mux1 : Mux  Inputs=2
  Product : Product  RndMeth=Zero
  Product1 : Product  RndMeth=Zero
  Product2 : Product  RndMeth=Zero
  Sin : Trigonometry
  Sum : Sum  Tag=Test  Inputs=++|
  Sum1 : Sum  Inputs=|-+
  Sum2 : Sum  Inputs=|+|
  Ter3 : Terminator  Commented=on
  Trigonometric Function : Trigonometry  Commented=on  Operator=atan2
  Fourier : Outport
  Phase : Outport  Port=2
  wires:
  fundamental frequency/1 -> Product1/1, Integrator1/1
  Integrator1/1 -> Gain3/1
  Gain3/1 -> Sin/1
  Demux2/1 -> Ter3/1
  Demux2/2 -> Demux1/1
  Gain2/1 -> Trigonometric Function/1
  Demux1/2 -> Gain2/1
  Demux1/1 -> Trigonometric Function/2
  Product/1 -> Integrator/1(u)
  Trigonometric Function/1 -> Phase/1
  Sum2/1 -> Sum1/1
  harmonic basis/1 -> Product2/1, Product/1
  input signal/1 -> Sum1/2
  Product2/1 -> Sum2/1
  Sum1/1 -> Product/2
  Latched first order hold/1(Out) -> Sum/1
  Sum/1 -> Demux2/1, Fourier/1, Latched first order hold/1(In), Product2/2
  Data Type Conversion1/1 -> Sum/2
  Mux1/1 -> Data Type Conversion1/1
  First order hold/1(Out) -> Demux/1
  Demux/2 -> Mux1/2
  Gain1/1 -> Mux1/1
  Demux/1 -> Gain1/1
  Integrator/1(int) -> Gain/1
  Sin/1 -> Latched first order hold/Trigger, First order hold/Trigger, Integrator/2(reset)
  Gain/1 -> Product1/2
  Product1/1 -> First order hold/1(In)

== system model1/RTF_estimator4/Subsystem/Harmonic Basis Gen1 ==
  fund_freq : Inport
  Cos : Trigonometry  Operator=cos
  DC : Constant
  Gain1 : Gain  Gain=2*pi
  Integrator : Integrator
  Mux : Mux  Inputs=3
  Product : Product
  Sin : Trigonometry
  harmonics_array : Constant  Value=1:k_harmonics
  harmonic_basis : Outport  OutDataTypeStr=double  SampleTime=0
  wires:
  Gain1/1 -> Sin/1, Cos/1
  Mux/1 -> harmonic_basis/1
  Integrator/1 -> Product/1
  Cos/1 -> Mux/2
  Product/1 -> Gain1/1
  Sin/1 -> Mux/3
  harmonics_array/1 -> Product/2
  fund_freq/1 -> Integrator/1
  DC/1 -> Mux/1

== system model1/RTF_estimator1/Subsystem/Fourier Series 2/First order hold ==
  In : Inport  LatchByDelayingOutsideSignal=on
  Trigger : TriggerPort  VariantControl=(inherit)
  Out : Outport
  wires:
  In/1 -> Out/1

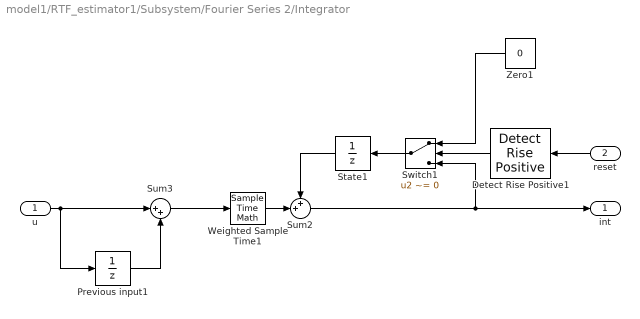
== system model1/RTF_estimator1/Subsystem/Fourier Series 2/Integrator ==
  u : Inport
  reset : Inport  Port=2
  Detect Rise Positive1 : simulink/Logic and Bit Operations/Detect Rise Positive  vinit=0  OutDataTypeStr=uint8
  Previous input1 : UnitDelay  SampleTime=-1  HasFrameUpgradeWarning=on
  State1 : UnitDelay  SampleTime=-1  HasFrameUpgradeWarning=on
  Sum2 : Sum  Inputs=++|
  Sum3 : Sum  Inputs=|++
  Switch1 : Switch  Criteria=u2 ~= 0  SaturateOnIntegerOverflow=off  InputSameDT=off
  Weighted Sample Time1 : SampleTimeMath  TsampMathOp=*  weightValue=0.5
  Zero1 : Constant  Value=0
  int : Outport
  wires:
  State1/1 -> Sum2/1
  Sum2/1 -> Switch1/3, int/1
  Weighted Sample Time1/1 -> Sum2/2
  Sum3/1 -> Weighted Sample Time1/1
  u/1 -> Sum3/1, Previous input1/1
  Previous input1/1 -> Sum3/2
  reset/1 -> Detect Rise Positive1/1
  Switch1/1 -> State1/1
  Zero1/1 -> Switch1/1
  Detect Rise Positive1/1 -> Switch1/2

== system model1/RTF_estimator1/Subsystem/Fourier Series 2/Latched first order hold ==
  In : Inport  LatchByDelayingOutsideSignal=on
  Trigger : TriggerPort  VariantControl=(inherit)
  Out : Outport
  wires:
  In/1 -> Out/1

== system model1/RTF_estimator2/Subsystem/Fourier Series 2/First order hold ==
  In : Inport  LatchByDelayingOutsideSignal=on
  Trigger : TriggerPort  VariantControl=(inherit)
  Out : Outport
  wires:
  In/1 -> Out/1

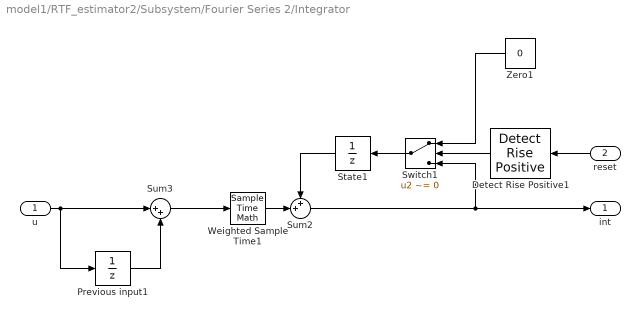
== system model1/RTF_estimator2/Subsystem/Fourier Series 2/Integrator ==
  u : Inport
  reset : Inport  Port=2
  Detect Rise Positive1 : simulink/Logic and Bit Operations/Detect Rise Positive  vinit=0  OutDataTypeStr=uint8
  Previous input1 : UnitDelay  SampleTime=-1  HasFrameUpgradeWarning=on
  State1 : UnitDelay  SampleTime=-1  HasFrameUpgradeWarning=on
  Sum2 : Sum  Inputs=++|
  Sum3 : Sum  Inputs=|++
  Switch1 : Switch  Criteria=u2 ~= 0  SaturateOnIntegerOverflow=off  InputSameDT=off
  Weighted Sample Time1 : SampleTimeMath  TsampMathOp=*  weightValue=0.5
  Zero1 : Constant  Value=0
  int : Outport
  wires:
  Detect Rise Positive1/1 -> Switch1/2
  Zero1/1 -> Switch1/1
  Switch1/1 -> State1/1
  reset/1 -> Detect Rise Positive1/1
  Previous input1/1 -> Sum3/2
  u/1 -> Previous input1/1, Sum3/1
  Sum3/1 -> Weighted Sample Time1/1
  Weighted Sample Time1/1 -> Sum2/2
  Sum2/1 -> int/1, Switch1/3
  State1/1 -> Sum2/1

== system model1/RTF_estimator2/Subsystem/Fourier Series 2/Latched first order hold ==
  In : Inport  LatchByDelayingOutsideSignal=on
  Trigger : TriggerPort  VariantControl=(inherit)
  Out : Outport
  wires:
  In/1 -> Out/1

== system model1/RTF_estimator4/Subsystem/Fourier Series 2/First order hold ==
  In : Inport  LatchByDelayingOutsideSignal=on
  Trigger : TriggerPort  VariantControl=(inherit)
  Out : Outport
  wires:
  In/1 -> Out/1

== system model1/RTF_estimator4/Subsystem/Fourier Series 2/Integrator ==
  u : Inport
  reset : Inport  Port=2
  Detect Rise Positive1 : simulink/Logic and Bit Operations/Detect Rise Positive  vinit=0  OutDataTypeStr=uint8
  Previous input1 : UnitDelay  SampleTime=-1  HasFrameUpgradeWarning=on
  State1 : UnitDelay  SampleTime=-1  HasFrameUpgradeWarning=on
  Sum2 : Sum  Inputs=++|
  Sum3 : Sum  Inputs=|++
  Switch1 : Switch  Criteria=u2 ~= 0  SaturateOnIntegerOverflow=off  InputSameDT=off
  Weighted Sample Time1 : SampleTimeMath  TsampMathOp=*  weightValue=0.5
  Zero1 : Constant  Value=0
  int : Outport
  wires:
  State1/1 -> Sum2/1
  Sum2/1 -> Switch1/3, int/1
  Weighted Sample Time1/1 -> Sum2/2
  Sum3/1 -> Weighted Sample Time1/1
  u/1 -> Sum3/1, Previous input1/1
  Previous input1/1 -> Sum3/2
  reset/1 -> Detect Rise Positive1/1
  Switch1/1 -> State1/1
  Zero1/1 -> Switch1/1
  Detect Rise Positive1/1 -> Switch1/2

== system model1/RTF_estimator4/Subsystem/Fourier Series 2/Latched first order hold ==
  In : Inport  LatchByDelayingOutsideSignal=on
  Trigger : TriggerPort  VariantControl=(inherit)
  Out : Outport
  wires:
  In/1 -> Out/1

== matlab function model1/MATLAB Function3 ==
  data: Coeffs input; avgCoeffs output
function avgCoeffs = exponentialAverage(Coeffs)
% Smooth Fourier coefficients using exponential moving average (EMA)

% Tuning parameter
alpha = 1e-7;  % Adjust between 0.001 (slow) to 0.1 (fast)

% Persistent storage
persistent avg
if isempty(avg)
    avg = Coeffs;
end

% Update rule
avg = alpha * Coeffs + (1 - alpha) * avg;

% Output
avgCoeffs = avg;

== matlab function model1/duffing/MATLAB Function ==
  data: x input; dxdt output; v input; excitation input; dvdt output
function [dxdt, dvdt] = duffingDerivatives(x, v, excitation)
% Duffing oscillator derivatives
%
% Inputs:
%   x - displacement
%   v - velocity
%   excitation - external excitation signal
%
% Outputs:
%   dx/dt dv/dt

% Define Duffing parameters

% stable duffing
delta = 0.2;    % damping
alpha = +1;     % linear stiffness
beta  = 1;      % nonlinear stiffness

% bi-stable duffing
% delta = 0.2;    % damping
% alpha = -1;     % linear stiffness
% beta  = 1;      % nonlinear stiffness

% bi-stable duffing from Rezaee, Renson: https://doi.org/10.1137/23M1587774
% delta = 0.1;    % damping
% alpha = -4;     % linear stiffness
% beta  = 2;      % nonlinear stiffness


% Duffing equation derivatives
dxdt = v;
dvdt = excitation - delta*v - alpha*x - beta*x^3;

end

== matlab function model1/RTF_estimator2/MATLAB Function2 ==
  data: Coeffs input; avgCoeffs output
function avgCoeffs = exponentialAverage(Coeffs)
% Smooth Fourier coefficients using exponential moving average (EMA)

% Tuning parameter
alpha = 5e-5;  % Adjust between 0.001 (slow) to 0.1 (fast)

% Persistent storage
persistent avg
if isempty(avg)
    avg = Coeffs;
end

% Update rule
avg = alpha * Coeffs + (1 - alpha) * avg;

% Output
avgCoeffs = avg;

== matlab function model1/RTF_estimator2/MATLAB Function3 ==
  data: Coeffs input; avgCoeffs output
function avgCoeffs = exponentialAverage(Coeffs)
% Smooth Fourier coefficients using exponential moving average (EMA)

% Tuning parameter
alpha = 0.0005;  % Adjust between 0.001 (slow) to 0.1 (fast)

% Persistent storage
persistent avg
if isempty(avg)
    avg = Coeffs;
end

% Update rule
avg = alpha * Coeffs + (1 - alpha) * avg;

% Output
avgCoeffs = avg;

== matlab function model1/duffing1/MATLAB Function ==
  data: x input; dxdt output; v input; excitation input; dvdt output
function [dxdt, dvdt] = duffingDerivatives(x, v, excitation)
% Duffing oscillator derivatives
%
% Inputs:
%   x - displacement
%   v - velocity
%   excitation - external excitation signal
%
% Outputs:
%   dx/dt dv/dt

% Define Duffing parameters

% stable duffing
delta = 0.2;    % damping
alpha = +1;     % linear stiffness
beta  = 1;      % nonlinear stiffness

% bi-stable duffing
% delta = 0.2;    % damping
% alpha = -1;     % linear stiffness
% beta  = 1;      % nonlinear stiffness

% bi-stable duffing from Rezaee, Renson: https://doi.org/10.1137/23M1587774
% delta = 0.1;    % damping
% alpha = -4;     % linear stiffness
% beta  = 2;      % nonlinear stiffness


% Duffing equation derivatives
dxdt = v;
dvdt = excitation - delta*v - alpha*x - beta*x^3;

end

== matlab function model1/MATLAB Function2 ==
  data: Coeffs input; avgCoeffs output
function avgCoeffs = exponentialAverage(Coeffs)
% Smooth Fourier coefficients using exponential moving average (EMA)

% Tuning parameter
alpha = 5e-5;  % Adjust between 0.001 (slow) to 0.1 (fast)

% Persistent storage
persistent avg
if isempty(avg)
    avg = Coeffs;
end

% Update rule
avg = alpha * Coeffs + (1 - alpha) * avg;

% Output
avgCoeffs = avg;

== matlab function model1/MATLAB Function1 ==
  data: Coeffs input; avgCoeffs output
function avgCoeffs = exponentialAverage(Coeffs)
% Smooth Fourier coefficients using exponential moving average (EMA)

% Tuning parameter
alpha = 1e-6;  % Adjust between 0.001 (slow) to 0.1 (fast)

% Persistent storage
persistent avg
if isempty(avg)
    avg = Coeffs;
end

% Update rule
avg = alpha * Coeffs + (1 - alpha) * avg;

% Output
avgCoeffs = avg;

== matlab function model1/RTF_estimator1/MATLAB Function1 ==
  data: Coeffs input; avgCoeffs output; varCoeffs output
function [avgCoeffs, varCoeffs] = exponentialAverageWithVariance(Coeffs)
% Exponential Moving Average (EMA) and Variance (EMV) for Fourier Coefficients

% Tuning parameter
alpha = 5e-4;  % 0.001 (slow, smooth) to 0.1 (fast, responsive)

% Persistent storage
persistent avg sqAvg
if isempty(avg)
    avg = Coeffs;
    sqAvg = Coeffs.^2;
end

% EMA update
avg = alpha * Coeffs + (1 - alpha) * avg;

% EMA of square
sqAvg = alpha * (Coeffs.^2) + (1 - alpha) * sqAvg;

% Variance = E[x^2] - (E[x])^2
varCoeffs = sqAvg - avg.^2;

% Output
avgCoeffs = avg;
end

== matlab function model1/RTF_estimator4/MATLAB Function1 ==
  data: Coeffs input; avgCoeffs output; varCoeffs output
function [avgCoeffs, varCoeffs] = exponentialAverageWithVariance(Coeffs)
% Exponential Moving Average (EMA) and Variance (EMV) for Fourier Coefficients

% Tuning parameter
alpha = 5e-4;  % 0.001 (slow, smooth) to 0.1 (fast, responsive)

% Persistent storage
persistent avg sqAvg
if isempty(avg)
    avg = Coeffs;
    sqAvg = Coeffs.^2;
end

% EMA update
avg = alpha * Coeffs + (1 - alpha) * avg;

% EMA of square
sqAvg = alpha * (Coeffs.^2) + (1 - alpha) * sqAvg;

% Variance = E[x^2] - (E[x])^2
varCoeffs = sqAvg - avg.^2;

% Output
avgCoeffs = avg;
end
